simulink model "calcparam"  (R2019a)
settings: Solver=VariableStepAuto  StartTime=0.0  StopTime=160  RelTol=1e-3
values from neighbouring files (symbols this model uses):
  d = 0.01    [workspace.mat]
  Q = 31.2    [workspace.mat]
undefined symbols (not defined in the file or in its folder): c1, r0, r1, soc_1
libraries: simulink x2
settings Model: Creator=sujan  LastModifiedBy=sujan

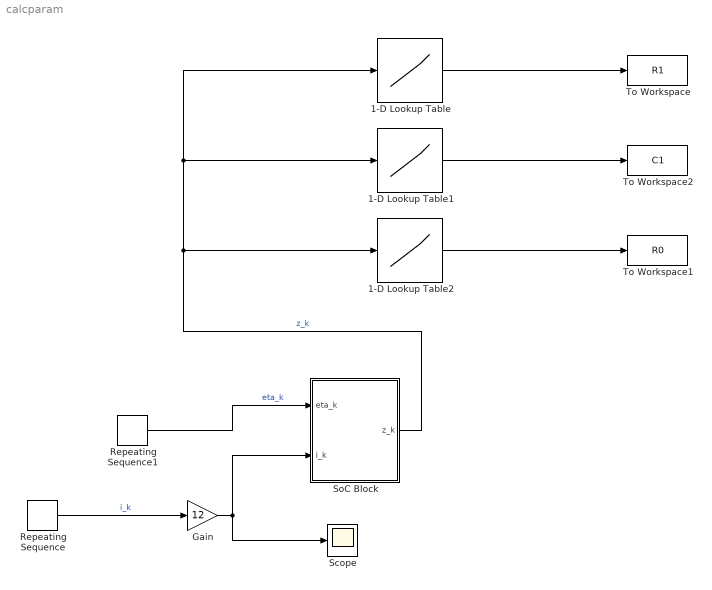
== system calcparam ==
  1-D Lookup Table : Lookup_n-D  NumberOfTableDimensions=1  BreakpointsForDimension1=soc_1.soc_1  Table=r1.r1  InternalRulePriority=Speed  RndMeth=Simplest  InputSameDT=on
  1-D Lookup Table1 : Lookup_n-D  NumberOfTableDimensions=1  BreakpointsForDimension1=soc_1.soc_1  Table=c1.c1  InternalRulePriority=Speed  RndMeth=Simplest  InputSameDT=on
  1-D Lookup Table2 : Lookup_n-D  NumberOfTableDimensions=1  BreakpointsForDimension1=soc_1.soc_1  Table=r0.r0  InternalRulePriority=Speed  RndMeth=Simplest  InputSameDT=on
  Gain : Gain  Gain=12
  Repeating Sequence : simulink/Sources/Repeating Sequence  rep_seq_t=time  rep_seq_y=I
  Repeating Sequence1 : simulink/Sources/Repeating Sequence  rep_seq_t=time  rep_seq_y=eta1
  Scope : Scope
  "SoC Block " : Subsystem
  To Workspace : ToWorkspace  VariableName=R1  SaveFormat=Timeseries  SampleTime=-1
      settings: Save2DSignal=2-D array (concatenate along first dimension)
  To Workspace1 : ToWorkspace  VariableName=R0  SaveFormat=Timeseries  SampleTime=-1
      settings: Save2DSignal=2-D array (concatenate along first dimension)
  To Workspace2 : ToWorkspace  VariableName=C1  SaveFormat=Timeseries  SampleTime=-1
      settings: Save2DSignal=2-D array (concatenate along first dimension)
  wires:
  1-D Lookup Table/1 -> To Workspace/1
  1-D Lookup Table1/1 -> To Workspace2/1
  1-D Lookup Table2/1 -> To Workspace1/1
  "SoC Block "/1(z_k) -> 1-D Lookup Table/1, 1-D Lookup Table1/1, 1-D Lookup Table2/1  "z_k"
  Repeating Sequence1/1 -> "SoC Block "/1(eta_k)  "eta_k"
  Gain/1 -> "SoC Block "/2(i_k), Scope/1
  Repeating Sequence/1 -> Gain/1  "i_k"

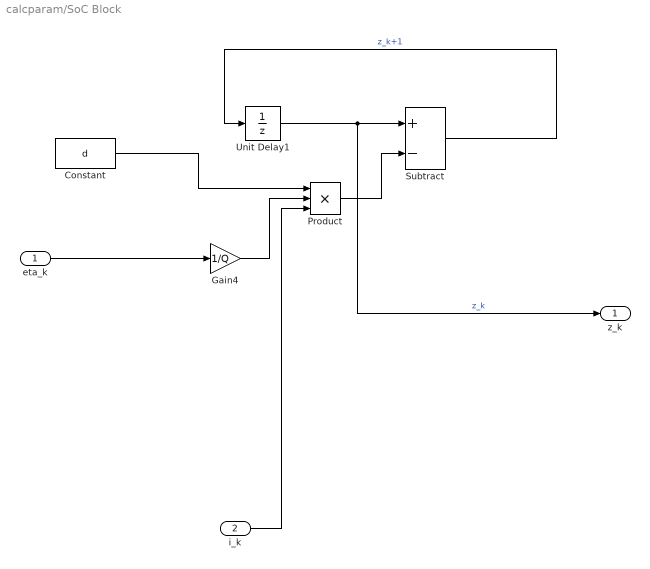
== system calcparam/SoC Block  ==
  eta_k : Inport
  i_k : Inport  Port=2
  Constant : Constant  Value=d
  Gain4 : Gain  Gain=1/Q
  Product : Product  Inputs=3
  Subtract : Sum  Inputs=+-
  Unit Delay1 : UnitDelay  InitialCondition=100  HasFrameUpgradeWarning=on
  z_k : Outport
  wires:
  Product/1 -> Subtract/2
  Constant/1 -> Product/1
  Unit Delay1/1 -> z_k/1, Subtract/1  "z_k"
  eta_k/1 -> Gain4/1
  Gain4/1 -> Product/2
  i_k/1 -> Product/3
  Subtract/1 -> Unit Delay1/1  "z_k+1"
